simulink model "ISC_V2"  (R2017b)
settings: Solver=VariableStepAuto  StartTime=0.0  StopTime=10.0  RelTol=1e-3
values from neighbouring files (symbols this model uses):
  du = 25    [main.m]
  p_a = 10^5    (= 100000)    [main.m]
  p_e = 1.2*10^5    (= 120000)    [main.m]
  theta_a = 295    [main.m]
  theta_m = 295    [main.m]
  ualpha = 5    [main.m]
undefined symbols (not defined in the file or in its folder): par
settings Model: Creator=gdgra  LastModifiedBy=gdgra

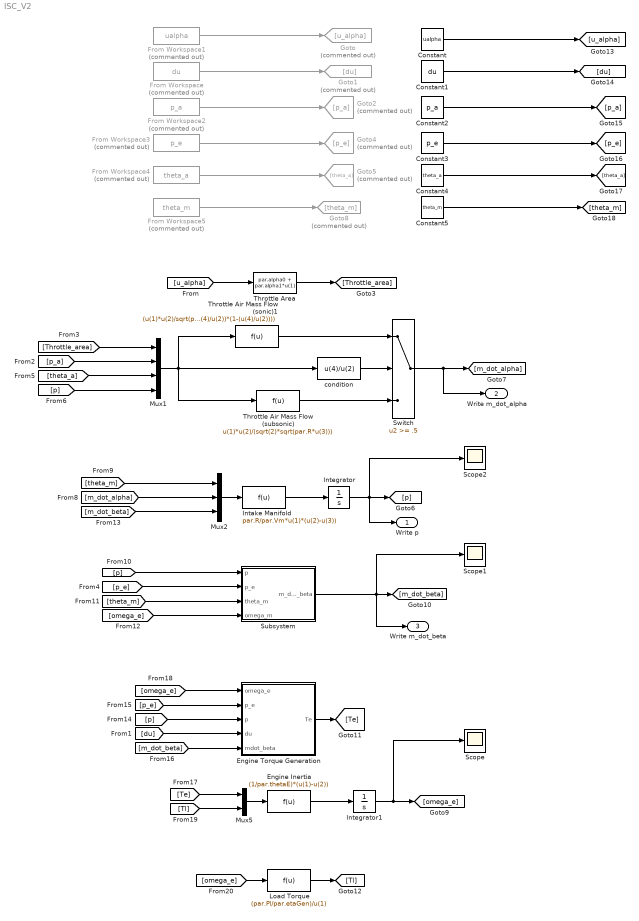
== system ISC_V2 ==
  Constant : Constant  Value=ualpha
  Constant1 : Constant  Value=du
  Constant2 : Constant  Value=p_a
  Constant3 : Constant  Value=p_e
  Constant4 : Constant  Value=theta_a
  Constant5 : Constant  Value=theta_m
  Engine Inertia : Fcn  Expr=(1/par.thetaE)*(u(1)-u(2))
  Engine Torque Generation : Subsystem
  From Workspace : FromWorkspace  Commented=on  VariableName=du  SampleTime=0
  From Workspace1 : FromWorkspace  Commented=on  VariableName=ualpha  SampleTime=0
  From Workspace2 : FromWorkspace  Commented=on  VariableName=p_a  SampleTime=0
  From Workspace3 : FromWorkspace  Commented=on  VariableName=p_e  SampleTime=0
  From Workspace4 : FromWorkspace  Commented=on  VariableName=theta_a  SampleTime=0
  From Workspace5 : FromWorkspace  Commented=on  VariableName=theta_m  SampleTime=0
  Goto : Goto  Commented=on  GotoTag=u_alpha
  Goto1 : Goto  Commented=on  GotoTag=du
  Goto2 : Goto  Commented=on  GotoTag=p_a
  Goto4 : Goto  Commented=on  GotoTag=p_e
  Goto5 : Goto  Commented=on  GotoTag=theta_a
  Goto8 : Goto  Commented=on  GotoTag=theta_m
  Intake Manifold : Fcn  Expr=par.R/par.Vm*u(1)*(u(2)-u(3))
  Integrator : Integrator  InitialCondition=p_a*.2
  Integrator1 : Integrator  InitialCondition=par.omegae0
  Load Torque : Fcn  Expr=(par.Pl/par.etaGen)/u(1)
  Mux1 : Mux
  Mux2 : Mux  Inputs=3
  Mux5 : Mux  Inputs=2
  Scope : Scope
  Scope1 : Scope
  Scope2 : Scope
  Subsystem : Subsystem
  Switch : Switch  Threshold=.5
  Throttle Air Mass Flow (sonic)1 : Fcn  Expr=(u(1)*u(2)/sqrt(par.R*u(3)))*sqrt(2*(u(4)/u(2))*(1-(u(4)/u(2))))
  Throttle Air Mass Flow (subsonic) : Fcn  Expr=u(1)*u(2)/(sqrt(2)*sqrt(par.R*u(3)))
  Throttle Area : Fcn  Expr=par.alpha0 + par.alpha1*u(1)
  "condition " : Fcn  Expr=u(4)/u(2)
  Write p : Outport
  Write m_dot_alpha : Outport  Port=2
  Write m_dot_beta : Outport  Port=3
  wires:
  From Workspace1/1 -> Goto/1
  From Workspace/1 -> Goto1/1
  From Workspace2/1 -> Goto2/1
  [u_alpha] -> Throttle Area/1
  Mux2/1 -> Intake Manifold/1
  Mux5/1 -> Engine Inertia/1
  Throttle Area/1 -> [Throttle_area]
  [Throttle_area] -> Mux1/1
  From Workspace3/1 -> Goto4/1
  From Workspace4/1 -> Goto5/1
  [p_a] -> Mux1/2
  [theta_a] -> Mux1/3
  Intake Manifold/1 -> Integrator/1
  Integrator/1 -> Scope2/1, Write p/1, [p]
  [p] -> Mux1/4
  Throttle Air Mass Flow (subsonic)/1 -> Switch/3
  Mux1/1 -> Throttle Air Mass Flow (sonic)1/1, Throttle Air Mass Flow (subsonic)/1, "condition "/1
  "condition "/1 -> Switch/2
  Throttle Air Mass Flow (sonic)1/1 -> Switch/1
  Switch/1 -> Write m_dot_alpha/1, [m_dot_alpha]
  [m_dot_alpha] -> Mux2/2
  From Workspace5/1 -> Goto8/1
  [theta_m] -> Mux2/1
  [p] -> Subsystem/1(p)
  [p_e] -> Subsystem/2(p_e)
  [theta_m] -> Subsystem/3(theta_m)
  Engine Inertia/1 -> Integrator1/1
  Integrator1/1 -> Scope/1, [omega_e]
  [omega_e] -> Subsystem/4(omega_m)
  Subsystem/1(m_dot_beta) -> Scope1/1, Write m_dot_beta/1, [m_dot_beta]
  [m_dot_beta] -> Mux2/3
  [m_dot_beta] -> Engine Torque Generation/5(mdot_beta)
  [du] -> Engine Torque Generation/4(du)
  [p] -> Engine Torque Generation/3(p)
  [p_e] -> Engine Torque Generation/2(p_e)
  Engine Torque Generation/1("Te ") -> [Te]
  [omega_e] -> Engine Torque Generation/1(omega_e)
  [Te] -> Mux5/1
  Load Torque/1 -> [Tl]
  [Tl] -> Mux5/2
  [omega_e] -> Load Torque/1
  Constant/1 -> [u_alpha]
  Constant1/1 -> [du]
  Constant2/1 -> [p_a]
  Constant3/1 -> [p_e]
  Constant4/1 -> [theta_a]
  Constant5/1 -> [theta_m]

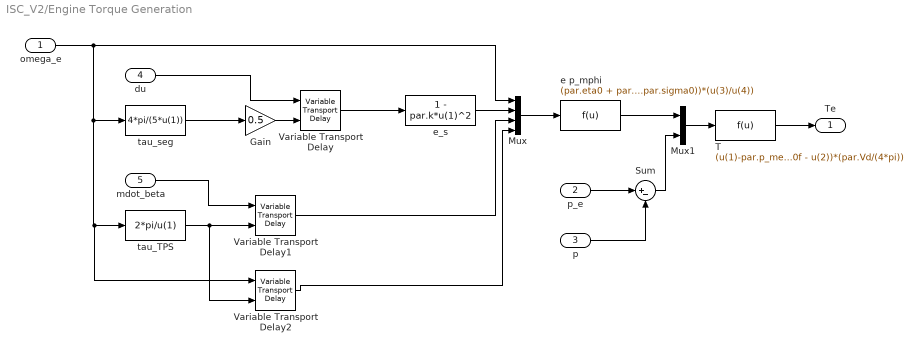
== system ISC_V2/Engine Torque Generation ==
  omega_e : Inport
  p_e : Inport  Port=2
  p : Inport  Port=3
  du : Inport  Port=4
  mdot_beta : Inport  Port=5
  Gain : Gain  Gain=0.5
  Mux : Mux
  Mux1 : Mux  Inputs=2
  Sum : Sum  Inputs=|+-
  T : Fcn  Expr=(u(1)-par.p_me0f - u(2))*(par.Vd/(4*pi))
  Variable Transport Delay : VariableTransportDelay  MaximumDelay=10  InitialOutput=du  MaximumPoints=10240
  Variable Transport Delay1 : VariableTransportDelay  MaximumDelay=10  InitialOutput=0.0044  MaximumPoints=10240
  Variable Transport Delay2 : VariableTransportDelay  MaximumDelay=10  InitialOutput=par.omegae0  MaximumPoints=10240
  e p_mphi : Fcn  Expr=(par.eta0 + par.eta1*u(1))*u(2)*(par.Hl/par.Vd)*(4*pi/(par.lambda*par.sigma0))*(u(3)/u(4))
  e_s : Fcn  Expr=1 - par.k*u(1)^2
  tau_TPS : Fcn  Expr=2*pi/u(1)
  tau_seg : Fcn  Expr=4*pi/(5*u(1))
  "Te " : Outport
  wires:
  du/1 -> Variable Transport Delay/1
  tau_seg/1 -> Gain/1
  Mux1/1 -> T/1
  omega_e/1 -> Variable Transport Delay2/1, tau_TPS/1, tau_seg/1, Mux/1
  Variable Transport Delay1/1 -> Mux/3
  mdot_beta/1 -> Variable Transport Delay1/1
  Variable Transport Delay2/1 -> Mux/4
  tau_TPS/1 -> Variable Transport Delay2/2, Variable Transport Delay1/2
  p/1 -> Sum/2
  Gain/1 -> Variable Transport Delay/2
  p_e/1 -> Sum/1
  Sum/1 -> Mux1/2
  Mux/1 -> e p_mphi/1
  e_s/1 -> Mux/2
  e p_mphi/1 -> Mux1/1
  Variable Transport Delay/1 -> e_s/1
  T/1 -> "Te "/1

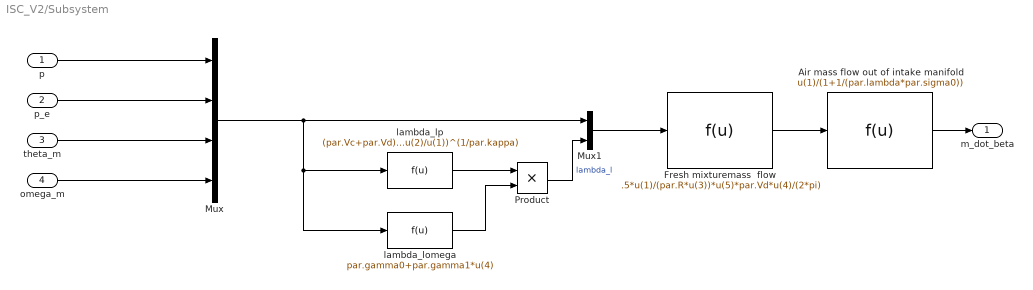
== system ISC_V2/Subsystem ==
  p : Inport
  p_e : Inport  Port=2
  theta_m : Inport  Port=3
  omega_m : Inport  Port=4
  Air mass flow out of intake manifold : Fcn  Expr=u(1)/(1+1/(par.lambda*par.sigma0))
  Fresh mixturemass  flow : Fcn  Expr=.5*u(1)/(par.R*u(3))*u(5)*par.Vd*u(4)/(2*pi)
  Mux : Mux
  Mux1 : Mux  Inputs=2
  Product : Product
  lambda_lomega : Fcn  Expr=par.gamma0+par.gamma1*u(4)
  lambda_lp : Fcn  Expr=(par.Vc+par.Vd)/par.Vd - (par.Vc/par.Vd)*(u(2)/u(1))^(1/par.kappa)
  m_dot_beta : Outport
  wires:
  p/1 -> Mux/1
  p_e/1 -> Mux/2
  theta_m/1 -> Mux/3
  omega_m/1 -> Mux/4
  Mux/1 -> lambda_lomega/1, lambda_lp/1, Mux1/1
  lambda_lp/1 -> Product/1
  lambda_lomega/1 -> Product/2
  Product/1 -> Mux1/2  "lambda_l"
  Mux1/1 -> Fresh mixturemass  flow/1
  Fresh mixturemass  flow/1 -> Air mass flow out of intake manifold/1
  Air mass flow out of intake manifold/1 -> m_dot_beta/1
